simulink model "Week1_Q2"  (R2020b)
settings: Solver=VariableStepAuto  StartTime=0.0  StopTime=10.0  RelTol=1e-3
settings Model: Creator=DELL  LastModifiedBy=DELL

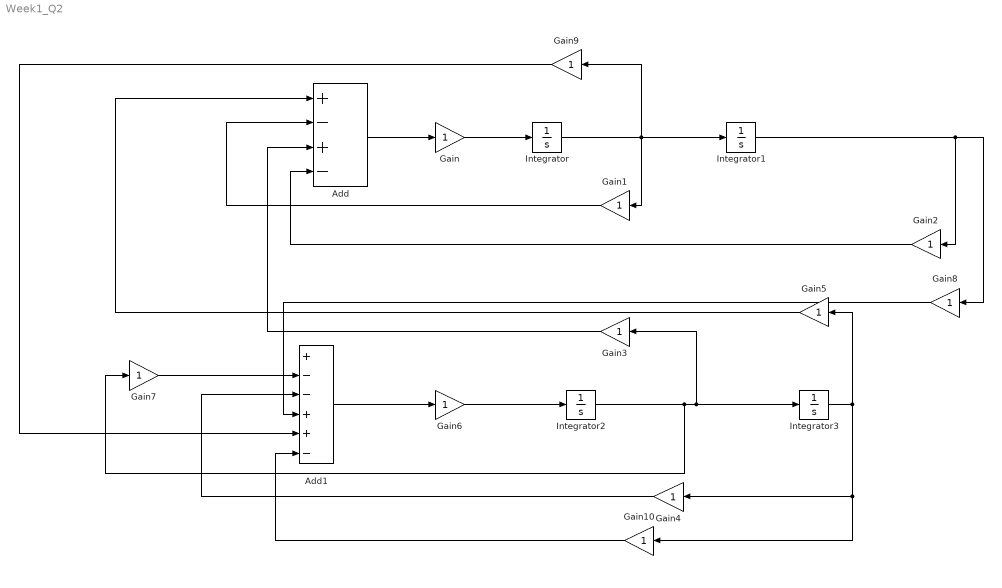
== system Week1_Q2 ==
  Add : Sum  Inputs=+-+-
  Add1 : Sum  Inputs=+--++-
  Gain{,1..10} (11 alike) : Gain
  Integrator{,1..3} (4 alike) : Integrator
  wires:
  Add/1 -> Gain/1
  Gain/1 -> Integrator/1
  Integrator/1 -> Gain9/1, Gain1/1, Integrator1/1
  Gain1/1 -> Add/2
  Integrator1/1 -> Gain8/1, Gain2/1
  Gain2/1 -> Add/4
  Add1/1 -> Gain6/1
  Gain6/1 -> Integrator2/1
  Integrator2/1 -> Gain7/1, Gain3/1, Integrator3/1
  Integrator3/1 -> Gain10/1, Gain4/1, Gain5/1
  Gain4/1 -> Add1/3
  Gain3/1 -> Add/3
  Gain5/1 -> Add/1
  Gain7/1 -> Add1/2
  Gain8/1 -> Add1/4
  Gain9/1 -> Add1/5
  Gain10/1 -> Add1/6
